simulink model "reservoirs"  (R2024b)
settings: Solver=ode45  StartTime=0.0  StopTime=30  MaxStep=0.05  RelTol=1e-3
libraries: simulink x2
settings Model: Creator=zv53855  LastModifiedBy=zv53855

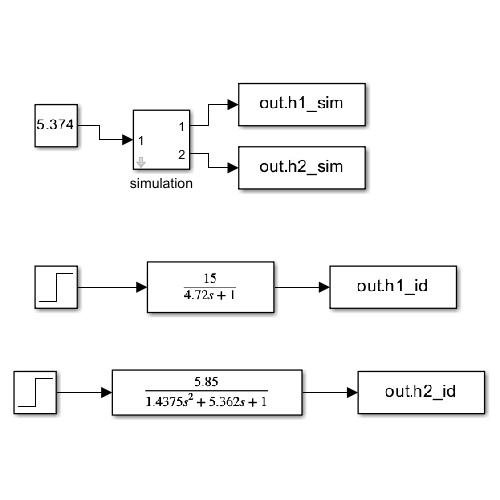
[thumbnail: Simulink's stored preview of the top-level diagram]
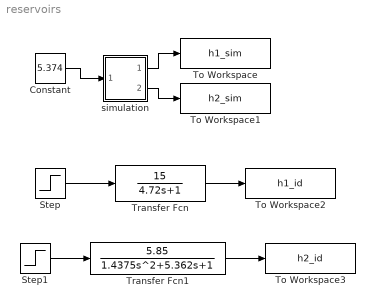
== system reservoirs ==
  Constant : Constant  Value=5.374
  Step : Step  Time=0  Before=1  SampleTime=0
  Step1 : Step  Time=0  Before=1  SampleTime=0
  To Workspace : ToWorkspace  VariableName=h1_sim  SaveFormat=Structure With Time  SampleTime=-1
  To Workspace1 : ToWorkspace  VariableName=h2_sim  SaveFormat=Structure With Time  SampleTime=-1
  To Workspace2 : ToWorkspace  VariableName=h1_id  SaveFormat=Structure With Time  SampleTime=-1
  To Workspace3 : ToWorkspace  VariableName=h2_id  SaveFormat=Structure With Time  SampleTime=-1
  Transfer Fcn : TransferFcn  Numerator=[15]  Denominator=[4.72 1]
  Transfer Fcn1 : TransferFcn  Numerator=[5.85]  Denominator=[1.4375, 5.362, 1]
  simulation : Subsystem  mask{h1_0=0, h2_0=0, S1=1, S2=0.5, Swy1=1, Swy2=0.5, phi1=0.4, phi2=1, g=9.81, Qwe=5.374}
      mask prompts: h1_0 "liquid level 1 init"; h2_0 "liquid level 2 init"; S1 "cross section reservoir 1"; S2 "cross section reservoir 2"; Swy1 "cross section outflow 1"; Swy2 "cross section outflow 2"; phi1 "coef 1"; phi2 "coef 2"; Qwe "liquid tributary"
  wires:
  Step/1 -> Transfer Fcn/1
  simulation/2(Out2) -> To Workspace1/1
  simulation/1(Out1) -> To Workspace/1
  Constant/1 -> simulation/1(In1)
  Transfer Fcn/1 -> To Workspace2/1
  Step1/1 -> Transfer Fcn1/1
  Transfer Fcn1/1 -> To Workspace3/1

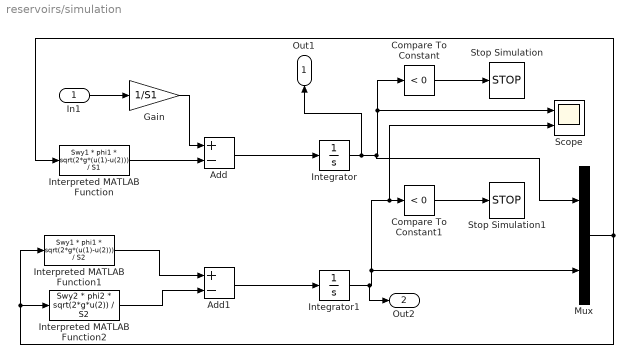
== system reservoirs/simulation ==
  In1 : Inport
  Add : Sum  Inputs=+-
  Add1 : Sum  Inputs=+-
  Compare To Constant : simulink/Logic and Bit Operations/Compare To Constant  relop=<  const=0  OutDataTypeStr=boolean
  Compare To Constant1 : simulink/Logic and Bit Operations/Compare To Constant  relop=<  const=0  OutDataTypeStr=boolean
  Gain : Gain  Gain=1/S1
  Integrator : Integrator  InitialCondition=h1_0
  Integrator1 : Integrator  InitialCondition=h2_0
  Interpreted MATLAB Function : MATLABFcn  MATLABFcn=Swy1 * phi1 * sqrt(2*g*(u(1)-u(2))) / S1
  Interpreted MATLAB Function1 : MATLABFcn  MATLABFcn=Swy1 * phi1 * sqrt(2*g*(u(1)-u(2))) / S2
  Interpreted MATLAB Function2 : MATLABFcn  MATLABFcn=Swy2 * phi2 * sqrt(2*g*u(2)) / S2
  Mux : Mux  Inputs=2
  Scope : Scope  NumInputPorts=2
  Stop Simulation : Stop
  Stop Simulation1 : Stop
  Out1 : Outport
  Out2 : Outport  Port=2
  wires:
  Compare To Constant/1 -> Stop Simulation/1
  Add/1 -> Integrator/1
  Integrator/1 -> Out1/1, Mux/1, Scope/1, Compare To Constant/1
  Gain/1 -> Add/1
  Interpreted MATLAB Function/1 -> Add/2
  Compare To Constant1/1 -> Stop Simulation1/1
  Integrator1/1 -> Out2/1, Mux/2, Scope/2, Compare To Constant1/1
  Add1/1 -> Integrator1/1
  Interpreted MATLAB Function1/1 -> Add1/1
  Interpreted MATLAB Function2/1 -> Add1/2
  Mux/1 -> Interpreted MATLAB Function2/1, Interpreted MATLAB Function1/1, Interpreted MATLAB Function/1
  In1/1 -> Gain/1
